simulink model "motor_ident"  (R2015a)
settings: Solver=ode1  StartTime=0.0  StopTime=420  FixedStep=0.002  RelTol=1e-3
undefined symbols (not defined in the file): HIL, sigbuilder_block
libraries: quarc_library x3, simulink_extras x1, simulink x1
settings Model: SimulationMode=external  ExtModeTrigDuration=10000  Creator=bemran  LastModifiedBy=bemran
settings SolverCC: PositivePriorityOrder=on
settings DataIOCC: MaxDataPoints=1000000  SignalLogging=off  DSMLogging=off
settings RTWCC: SystemTargetFile=quarc_win64.tlc  TemplateMakefile=quarc_default_tmf  Description=QUARC Win64 Target
settings STFCustomTargetCC: TargetLibSuffix=.lib  TargetPreCompLibLocation=C:\PROGRA~3\QUARC\lib\2015a\win64\release  GenerateSampleERTMain=off  ConcurrentExecutionCompliant=on  GeneratePreprocessorConditionals=Disable all  ERTCustomFileBanners=off  SupportNonInlinedSFcns=on  SupportVariableSizeSignals=off  MATLABClassNameForMDSCustomization=Simulink.SoftwareTarget.GRTCustomization  GRTInterface=on  SystemTargetFile=quarc_win64.tlc
settings GRTTargetCC: TargetPreCompLibLocation=C:\PROGRA~3\QUARC\lib\2015a\win64\release  ParMdlRefBuildCompliant=off  CompOptLevelCompliant=off  CombineOutputUpdateFcns=off  MatFileLogging=off  CPPClassGenCompliant=off  GRTInterface=on  ExtMode=on  ExtModeMexFile=quarc_comm

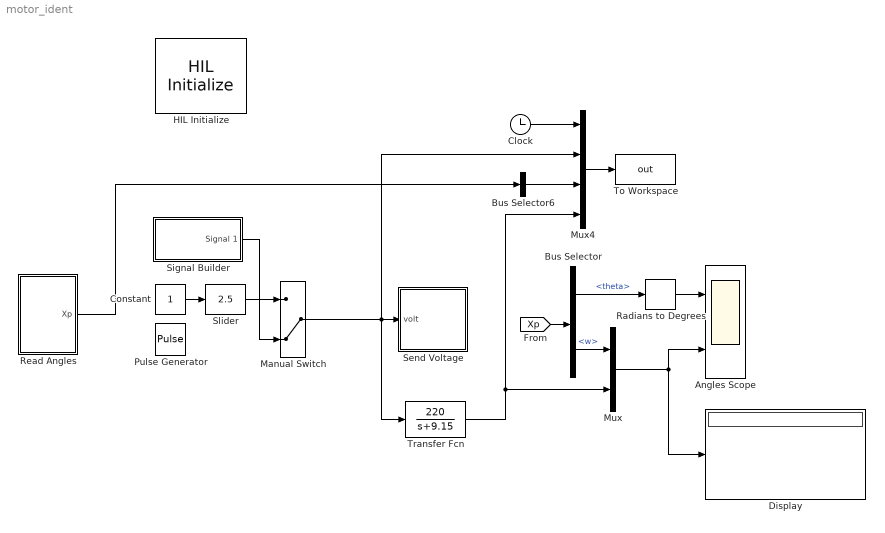
== system motor_ident ==
  Angles Scope : Scope  NumInputPorts=2
      settings: TimeRange=100  YMin=43000~-100  YMax=50000~100  SaveName=ScopeData2
  Bus Selector : BusSelector  OutputSignals=theta,w
  Bus Selector6 : BusSelector  OutputSignals=theta  OutputAsBus=on
  Clock : Clock
  Constant : Constant
  Display : Display
  HIL Initialize : quarc_library/Data Acquisition/Generic/Configuration/HIL Initialize  Priority=-99  object_name=HIL-1  board_type=qube_servo2_usb  board_number=0  board_options=""  exclusive=off  active=off  hardware_clocks=[0]  clock_modes=[]  initial_clock_frequencies=[]  set_clock_params_at_start=off  set_clock_params_at_switch_in=off  set_clock_frequencies_at_start=off  set_clock_frequencies_at_switch_in=off  analog_input_channels=[0]  analog_input_maximums=3  analog_input_minimums=-3  set_analog_input_params_at_start=off  set_analog_input_params_at_switch_in=off  analog_output_channels=[0]  analog_output_maximums=15  analog_output_minimums=-15  initial_analog_outputs=[0]  final_analog_outputs=[0]  watchdog_analog_outputs=0  set_analog_output_params_at_start=off  set_analog_output_params_at_switch_in=off  set_analog_outputs_at_start=on  set_analog_outputs_at_switch_in=off  set_analog_outputs_at_terminate=on  set_analog_outputs_at_switch_out=off  set_analog_outputs_on_watchdog=on  digital_input_channels=[]  digital_output_channels=[0]  digital_output_configuration=[]  initial_digital_outputs=[1]  final_digital_outputs=[0]  watchdog_digital_outputs=[0]  set_digital_output_params_at_start=off  set_digital_output_params_at_switch_in=off  set_digital_outputs_at_start=on  set_digital_outputs_at_switch_in=off  set_digital_outputs_at_terminate=on  set_digital_outputs_at_switch_out=off  set_digital_outputs_on_watchdog=on  encoder_channels=[0:1]  quadrature=[4]  encoder_filter_frequency=[]  initial_encoder_counts=[0]  set_encoder_params_at_start=off  set_encoder_params_at_switch_in=off  set_encoder_counts_at_start=on  set_encoder_counts_at_switch_in=off  pwm_channels=[]  pwm_modes=[]  pwm_frequency=[]  pwm_configuration=[]  pwm_alignment=[]  pwm_polarity=[]  pwm_leading_deadband=[]  pwm_trailing_deadband=[]  initial_pwm_outputs=[]  final_pwm_outputs=[]  watchdog_pwm_outputs=[]  set_pwm_params_at_start=off  set_pwm_params_at_switch_in=off  set_pwm_outputs_at_start=off  set_pwm_outputs_at_switch_in=off  set_pwm_outputs_at_terminate=off  set_pwm_outputs_at_switch_out=off  set_pwm_outputs_on_watchdog=off  other_output_channels=[11000:11002]  initial_other_outputs=[0 1 0]  final_other_outputs=[1 0 0]  watchdog_other_outputs=[0 0 1]  set_other_outputs_at_start=on  set_other_outputs_at_switch_in=off  set_other_outputs_at_terminate=on  set_other_outputs_at_switch_out=off  set_other_outputs_on_watchdog=on
  Manual Switch : ManualSwitch  CurrentSetting=0
  Mux : Mux  Inputs=2
  Mux4 : Mux
  Pulse Generator : DiscretePulseGenerator  PulseType=Time based  Period=5  PulseWidth=50
  Radians to Degrees : simulink_extras/Transformations/Radians to Degrees
  Read Angles : Subsystem
  Send Voltage : Subsystem
  Signal Builder : Subsystem  Tag=STV Subsys  LoadFcn=sigbuilder_block('load');  StartFcn=sigbuilder_block('start');  StopFcn=sigbuilder_block('stop');  ClipboardFcn=sigbuilder_block('clipboard');  mask(Sigbuilder block){}
      mask help: Simulink:masks:SigbuilderBlock_MD
      mask init:
      | if ~strcmp(get_param(bdroot(gcbh),'SimulationStatus'),'stopped') tuvar = sigbuilder_block('maskInit'); end
      settings: CopyFcn=sigbuilder_block('copy');  DeleteFcn=sigbuilder_block('delete');  ModelCloseFcn=sigbuilder_block('modelClose');  PreSaveFcn=sigbuilder_block('preSave');  PauseFcn=sigbuilder_block('pause');  ContinueFcn=sigbuilder_block('continue');  NameChangeFcn=sigbuilder_block('namechange');  OpenFcn=sigbuilder_block('open',[437.6 199.2 550.4 400 ]);  CloseFcn=sigbuilder_block('close');
      mask Display: plot(0, 0, 100, 100,[2, 2, 32, 32, 2], [68, 8, 8, 68, 68],[32, 2], [38, 38], [32, 19, 2],[53, 60, 44], [32, 17, 17, 2],[16, 16, 31, 31]);txt = getActiveGroup(gcbh);text(2, 100, txt,'verticalAlignment', 'top');
  Slider : simulink/Math Operations/Slider Gain  low=0  gain=2.5  high=5
  To Workspace : ToWorkspace  VariableName=out  SampleTime=-1
  Transfer Fcn : TransferFcn  Numerator=[220]  Denominator=[1 9.15]
  wires:
  Bus Selector/1 -> Radians to Degrees/1  "<theta>"
  Radians to Degrees/1 -> Angles Scope/1
  Read Angles/1(Xp) -> Bus Selector6/1
  Bus Selector/2 -> Mux/1  "<w>"
  [Xp] -> Bus Selector/1
  Slider/1 -> Manual Switch/1
  Signal Builder/1(Signal 1) -> Manual Switch/2
  Manual Switch/1 -> Transfer Fcn/1, Mux4/2, Send Voltage/1(volt)
  Bus Selector6/1 -> Mux4/3
  Clock/1 -> Mux4/1
  Mux4/1 -> To Workspace/1
  Constant/1 -> Slider/1
  Transfer Fcn/1 -> Mux4/4, Mux/2
  Mux/1 -> Display/1, Angles Scope/2

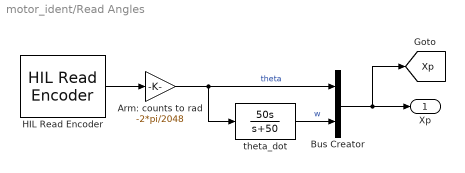
== system motor_ident/Read Angles ==
  Arm: counts to rad : Gain  Gain=-2*pi/2048
  Bus Creator : BusCreator  Inputs=2
  HIL Read Encoder : quarc_library/Data Acquisition/Generic/Immediate I//O/HIL Read Encoder  object_name=HIL-1  channels=0  sample_time=qc_get_step_size  active=on  vector_output=off  data_type_mode=Inherit via back propagation  data_type=double
  theta_dot : TransferFcn  Numerator=[50 0]  Denominator=[1 50]
  Xp : Outport
  tag scope: Xp=global
  wires:
  Arm: counts to rad/1 -> theta_dot/1, Bus Creator/1  "theta"
  HIL Read Encoder/1 -> Arm: counts to rad/1
  Bus Creator/1 -> Xp/1, [Xp]
  theta_dot/1 -> Bus Creator/2  "w"

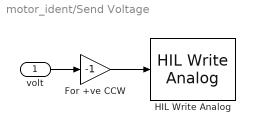
== system motor_ident/Send Voltage ==
  volt : Inport
  For +ve CCW : Gain  Gain=-1
  HIL Write Analog : quarc_library/Data Acquisition/Generic/Immediate I//O/HIL Write Analog  object_name=HIL-1  channels=0  sample_time=-1  active=off  vector_input=off
  wires:
  volt/1 -> For +ve CCW/1
  For +ve CCW/1 -> HIL Write Analog/1

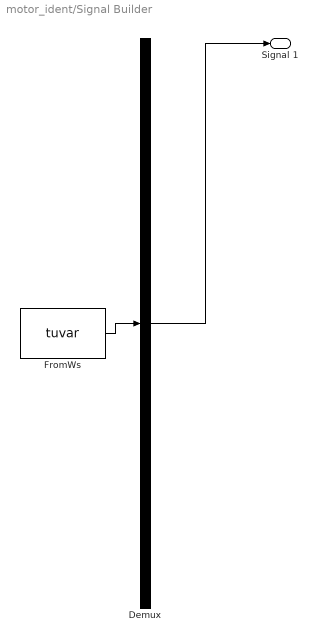
== system motor_ident/Signal Builder ==
  Demux : Demux  Tag=STV Demux  Outputs=1
  FromWs : FromWorkspace  Tag=STV FromWs  VariableName=tuvar  SampleTime=0
      SigBuilderData=|
      | common.afterFinalStr = 'Extrapolate'
      | common.sampleTime = 0
      | dataSet.timeRange = [0 500]
      | dataSet.name = 'Group 1'
      | sbobj.Groups.Name = 'Group 1'
      | sbobj.Groups.Signals.Name = 'Signal 1'
      | sbobj.Groups.Signals.XData = [0 10 10 20 20 30 30 40 40 50 50 60 60 70 70 80 80 90 90 100 100 110 110 120 120 130 130 140 140 150 150 160 160 170 170 180 180 190 190 200 200 210 210 220 220 230 230 240 240 250 250 260 260 270 270 280 280 290 290 300 300 310 310 320 320 330 330 340 340 350 350 360 360 370 370 380 380 390 390 400 400 410 410 420 420 430 430 440 440 450 450 460 460 470 470 480 480 490 490 500]
      | sbobj.Groups.Signals.YData = [0 0 -0.5 -0.5 0 0 0.5 0.5 0 0 -1 -1 0 0 1 1 0 0 -1.5 -1.5 0 0 1.5 1.5 0 0 -2 -2 0 0 2 2 0 0 -2.5 -2.5 0 0 2.5 2.5 0 0 -3 -3 0 0 3 3 0 0 -3.5 -3.5 0 0 3.5 3.5 0 0 -4 -4 0 0 4 4 0 0 -4.5 -4.5 0 0 4.5 4.5 0 0 -5 -5 0 0 5 5 0 0 -5 -5 0 0 5 5 2 2 -2 -2 2 2 -2 -2 1 1 -1 -1]
      | sbobj.Groups.TimeRange = [0 500]
  Signal 1 : Outport  Tag=STV Outport
  wires:
  Demux/1 -> Signal 1/1
  FromWs/1 -> Demux/1
